simulink model "Map_s"  (R2023a)
settings: Solver=VariableStepAuto  StartTime=0.0  StopTime=10.0  RelTol=1e-3
undefined symbols (not defined in the file): map_lead_den, map_lead_num, map_Ta_table, map_Tamax, map_Ts_bp, map_v_bp, Ts_ctrl
settings Model: Creator=Tan_Tram  LastModifiedBy=Tan_Tram

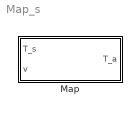
== system Map_s ==
  Map : Subsystem

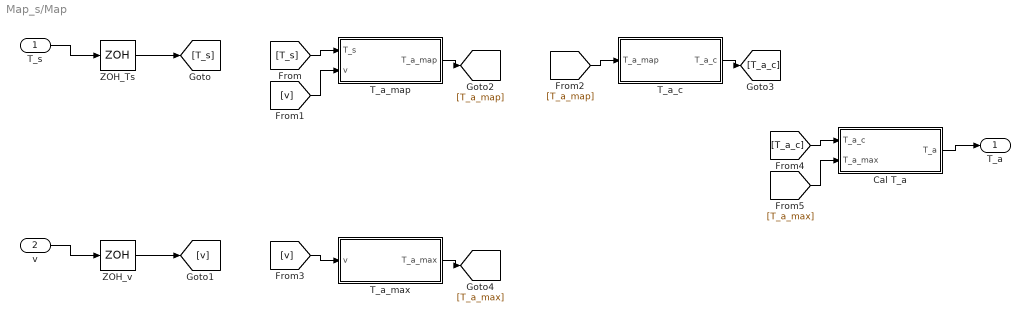
== system Map_s/Map ==
  T_s : Inport
  v : Inport  Port=2
  Cal T_a : Subsystem
  T_a_c : Subsystem
  T_a_map : Subsystem
  T_a_max : Subsystem
  ZOH_Ts : ZeroOrderHold  SampleTime=Ts_ctrl
  ZOH_v : ZeroOrderHold  SampleTime=Ts_ctrl
  T_a : Outport
  wires:
  T_s/1 -> ZOH_Ts/1
  v/1 -> ZOH_v/1
  ZOH_Ts/1 -> [T_s]
  ZOH_v/1 -> [v]
  [T_s] -> T_a_map/1(T_s)
  [v] -> T_a_map/2(v)
  T_a_map/1(T_a_map) -> [T_a_map]
  [T_a_map] -> T_a_c/1(T_a_map)
  T_a_c/1(T_a_c) -> [T_a_c]
  [v] -> T_a_max/1(v)
  T_a_max/1(T_a_max) -> [T_a_max]
  [T_a_c] -> Cal T_a/1(T_a_c)
  [T_a_max] -> Cal T_a/2(T_a_max)
  Cal T_a/1(T_a) -> T_a/1

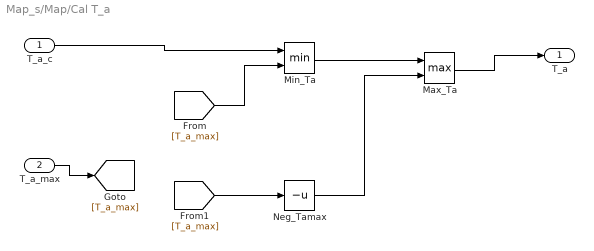
== system Map_s/Map/Cal T_a ==
  T_a_c : Inport
  T_a_max : Inport  Port=2
  Max_Ta : MinMax  Function=max  Inputs=2
  Min_Ta : MinMax  Inputs=2
  Neg_Tamax : UnaryMinus
  T_a : Outport
  wires:
  T_a_max/1 -> [T_a_max]
  T_a_c/1 -> Min_Ta/1
  [T_a_max] -> Min_Ta/2
  [T_a_max] -> Neg_Tamax/1
  Min_Ta/1 -> Max_Ta/1
  Neg_Tamax/1 -> Max_Ta/2
  Max_Ta/1 -> T_a/1

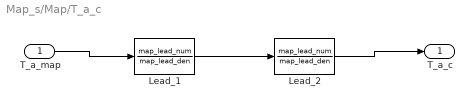
== system Map_s/Map/T_a_c ==
  T_a_map : Inport
  Lead_1 : DiscreteTransferFcn  Numerator=map_lead_num  Denominator=map_lead_den  SampleTime=Ts_ctrl
  Lead_2 : DiscreteTransferFcn  Numerator=map_lead_num  Denominator=map_lead_den  SampleTime=Ts_ctrl
  T_a_c : Outport
  wires:
  T_a_map/1 -> Lead_1/1
  Lead_1/1 -> Lead_2/1
  Lead_2/1 -> T_a_c/1

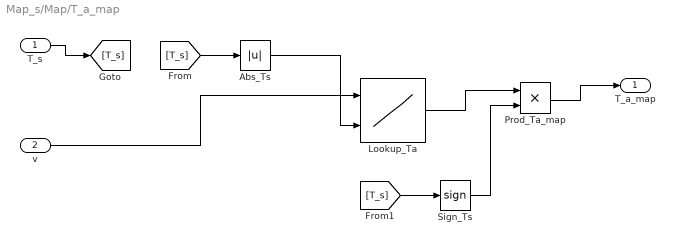
== system Map_s/Map/T_a_map ==
  T_s : Inport
  v : Inport  Port=2
  Abs_Ts : Abs  SaturateOnIntegerOverflow=off
  Lookup_Ta : Lookup_n-D  BreakpointsForDimension1=map_v_bp  BreakpointsForDimension2=map_Ts_bp  BreakpointsForDimension3=[5, 7]  Table=map_Ta_table  ExtrapMethod=Clip  InternalRulePriority=Speed  RndMeth=Simplest
      settings: InputPortMap=u0,u1
  Prod_Ta_map : Product  Inputs=**
  Sign_Ts : Signum
  T_a_map : Outport
  wires:
  T_s/1 -> [T_s]
  [T_s] -> Abs_Ts/1
  v/1 -> Lookup_Ta/1
  Abs_Ts/1 -> Lookup_Ta/2
  [T_s] -> Sign_Ts/1
  Lookup_Ta/1 -> Prod_Ta_map/1
  Sign_Ts/1 -> Prod_Ta_map/2
  Prod_Ta_map/1 -> T_a_map/1

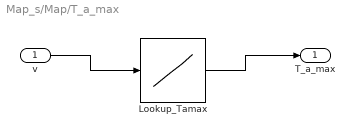
== system Map_s/Map/T_a_max ==
  v : Inport
  Lookup_Tamax : Lookup_n-D  NumberOfTableDimensions=1  BreakpointsForDimension1=map_v_bp  Table=map_Tamax  ExtrapMethod=Clip  InternalRulePriority=Speed  RndMeth=Simplest
  T_a_max : Outport
  wires:
  v/1 -> Lookup_Tamax/1
  Lookup_Tamax/1 -> T_a_max/1
